simulink model "integ_gain_slew_test"  (Simulink 6.6)
settings: Solver=ode45  StartTime=0.0  StopTime=10.0  RelTol=1e-3
undefined symbols (not defined in the file): alfa, gamma, GBW, slew, SR, Ts, VinHi
settings Model: Creator=yasuda  LastModifiedBy=yasuda

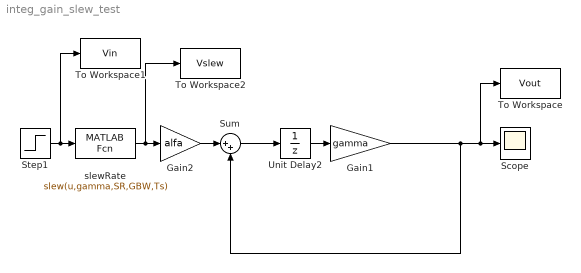
== system integ_gain_slew_test ==
  Gain1 : Gain  Gain=gamma
  Gain2 : Gain  Gain=alfa
  Scope : Scope
  Step1 : Step  After=VinHi  SampleTime=0
  Sum : Sum  Inputs=|++
  To Workspace : ToWorkspace  VariableName=Vout  SampleTime=1  SaveFormat=Array
  To Workspace1 : ToWorkspace  VariableName=Vin  SampleTime=1  SaveFormat=Array
  To Workspace2 : ToWorkspace  VariableName=Vslew  SampleTime=1  SaveFormat=Array
  Unit Delay2 : UnitDelay  SampleTime=Ts
  slewRate : MATLABFcn  MATLABFcn=slew(u,gamma,SR,GBW,Ts)
  wires:
  Sum/1 -> Unit Delay2/1
  Unit Delay2/1 -> Gain1/1
  Gain1/1 -> Sum/2, Scope/1, To Workspace/1
  Gain2/1 -> Sum/1
  slewRate/1 -> Gain2/1, To Workspace2/1
  Step1/1 -> slewRate/1, To Workspace1/1
